simulink model "APPL_PaFaultDetection"  (R2018b)
settings: configuration reference "CodeConfig_10_ms" (kept outside this file)
undefined symbols (not defined in the file): CAL_LockErrNoTime_30ms, CAL_ManualSwValid_90s, CAL_MotorHallInvalid_2s, CAL_MotorMaxRunTime_60s, CAL_MotorRelayErr_2s, CAL_MotorStall_750ms, D_DrSoftStopDef_B, D_DrSoftStopDef_F, D_DrSoftStopDef_H, D_DrSoftStopDef_L, D_Relay_DownBackFault, D_Relay_UpFrontFault, D_StallCurrent, enSeatMoveCmd, FALSE, TRUE
libraries: DareLib x91, simulink x2
(part 3 of 4)

== stateflow chart APPL_PaFaultDetection/LogicCtrl/HallError/HallErrorDetection ==
  note: #后期需要增加2F诊断判断20230510
  state MotorHallDetect
    state HeightHallError [parallel] [commented out]
      state Judge [commented out]
        ex:
        HeightHallTimer = 0;
        (default) -> (junction 286) [commented out]
        MotorHallDetect.HeightHallError.Judge -> (junction 286) [commented out]
        (junction 286) -> (junction 373) [commented out] : /*2s超时检测*/
            | [CAL_MotorHallInvalid_2s > HeightHallTimer]
        (junction 373) -> (junction 365) [commented out]
        (junction 286) -> (junction 262) [commented out] : {HeightHallTimer = CAL_MotorHallInvalid_2s;
            | HeightHallFault = 1;
            | Desc_HeightHallDTC = 1;}
        (junction 365) -> (junction 354) [commented out] : /* 粘连或无电机动作 */
            | [MtrCtrlFault_HeightUpVolt == MtrCtrlFault_HeightDownVolt ...
            | || enSeatMoveCmd.EN_NULL == MtrCtrlFault_HeightMotorCmd]
        (junction 365) -> (junction 381) [commented out] : {HeightHallTimer ++;}
        (junction 354) -> (junction 362) [commented out] : {HeightHallTimer = 0;}
        (junction 381) -> (junction 262) [commented out]
        (junction 362) -> (junction 381) [commented out]
        (junction 262) -> (junction 374) [commented out]
        (junction 374) -> (junction 261) [commented out] : /*霍尔计数变化*/
            | [hasChanged(MtrCtrlFault_HeightHallCnt)]
        (junction 374) -> (junction 357) [commented out]
        (junction 261) -> (junction 260) [commented out] : {HeightHallTimer = 0;
            | HeightHallFault = 0;
            | Desc_HeightHallDTC = 0;}
        (junction 260) -> (junction 357) [commented out]
      state Normal [commented out]
        en:
        HeightHallFault = 0;
      state Init [commented out]
        en:
        HeightHallFault = 0;
        Desc_HeightHallDTC = 0;
      (default) -> MotorHallDetect.HeightHallError.Normal [commented out]
      MotorHallDetect.HeightHallError.Normal -> MotorHallDetect.HeightHallError.Judge [commented out] : /*有调节动作*/
          | [enSeatMoveCmd.EN_NULL != MtrCtrlFault_HeightMotorCmd]
      MotorHallDetect.HeightHallError.Judge -> MotorHallDetect.HeightHallError.Normal [commented out] : /* */
          | [(hasChanged(HeightSwCmd) ...
          | || enSeatMoveCmd.EN_NULL == HeightSwCmd) ...
          | && enSeatMoveCmd.EN_NULL == MtrCtrlFault_HeightMotorCmd]
      MotorHallDetect.HeightHallError.Judge -> MotorHallDetect.HeightHallError.Init [commented out] : /* 不满足前置条件 */
          | [FALSE == DrAdj_Dtc_HeatingMat1SC]
      MotorHallDetect.HeightHallError.Init -> MotorHallDetect.HeightHallError.Normal [commented out] : /* 满足前置条件 */
          | [TRUE == DrAdj_Dtc_HeatingMat1SC]
      MotorHallDetect.HeightHallError.Normal -> MotorHallDetect.HeightHallError.Init [commented out] : /* 不满足前置条件 */
          | [FALSE == DrAdj_Dtc_HeatingMat1SC]
    state LengthHallError [parallel]
      settings: executionOrder=1
      state Normal
        en:
        LengthHallFault = 0;
      state Judge
        ex:
        LengthHallTimer = 0;
        (default) -> (junction 320)
        MotorHallDetect.LengthHallError.Judge -> (junction 320) [order 1]
        (junction 320) -> (junction 330) [order 1] : /*2s超时检测*/
            | [CAL_MotorHallInvalid_2s > LengthHallTimer]
        (junction 320) -> (junction 321) [order 2] : {LengthHallTimer = CAL_MotorHallInvalid_2s;
            | LengthHallFault = 1;
            | Desc_LengthHallDTC = 1;}
        (junction 330) -> (junction 401)
        (junction 401) -> (junction 382) [order 1] : /*粘连或无电机动作*/
            | [MtrCtrlFault_LengthForwardVolt == MtrCtrlFault_LengthBackwardVolt ...
            | || enSeatMoveCmd.EN_NULL == MtrCtrlFault_LengthMotorCmd]
        (junction 401) -> (junction 350) [order 2] : {LengthHallTimer ++;}
        (junction 382) -> (junction 372) : {LengthHallTimer = 0;}
        (junction 350) -> (junction 321)
        (junction 372) -> (junction 350)
        (junction 321) -> (junction 335)
        (junction 335) -> (junction 322) [order 1] : /*霍尔计数变化*/
            | [hasChanged(MtrCtrlFault_LengthHallCnt)]
        (junction 335) -> (junction 336) [order 2]
        (junction 322) -> (junction 323) : {LengthHallTimer = 0;
            | LengthHallFault = 0;
            | Desc_LengthHallDTC = 0;}
        (junction 323) -> (junction 336)
        (junction 336) -> (junction 361)
      state Init
        en:
        LengthHallFault = 0;
        Desc_LengthHallDTC = 0;
      (default) -> MotorHallDetect.LengthHallError.Normal
      MotorHallDetect.LengthHallError.Normal -> MotorHallDetect.LengthHallError.Judge [order 2] : /*有调节动作*/
          | [enSeatMoveCmd.EN_NULL != MtrCtrlFault_LengthMotorCmd]
      MotorHallDetect.LengthHallError.Judge -> MotorHallDetect.LengthHallError.Normal [order 2] : /*无调节动作*/
          | [(hasChanged(LengthSwCmd) ...
          | || enSeatMoveCmd.EN_NULL == LengthSwCmd) ...
          | && enSeatMoveCmd.EN_NULL == MtrCtrlFault_LengthMotorCmd]
      MotorHallDetect.LengthHallError.Judge -> MotorHallDetect.LengthHallError.Init [order 1] : /* 不满足前置条件 */
          | [FALSE == DrAdj_Dtc_HeatingMat1SC]
      MotorHallDetect.LengthHallError.Init -> MotorHallDetect.LengthHallError.Normal : /* 满足前置条件 */
          | [TRUE == DrAdj_Dtc_HeatingMat1SC]
      MotorHallDetect.LengthHallError.Normal -> MotorHallDetect.LengthHallError.Init [order 1] : /* 不满足前置条件 */
          | [FALSE == DrAdj_Dtc_HeatingMat1SC]
    state BackHallError [parallel]
      settings: executionOrder=2
      state Judge
        ex:
        BackHallTimer = 0;
        (default) -> (junction 398)
        MotorHallDetect.BackHallError.Judge -> (junction 398) [order 1]
        (junction 398) -> (junction 393) [order 1] : /*2s超时检测*/
            | [CAL_MotorHallInvalid_2s > BackHallTimer]
        (junction 398) -> (junction 387) [order 2] : {BackHallTimer = CAL_MotorHallInvalid_2s;
            | BackHallFault = 1;
            | Desc_BackHallDTC = 1;}
        (junction 393) -> (junction 367)
        (junction 367) -> (junction 355) [order 1] : /*粘连或无电机动作*/
            | [MtrCtrlFault_BackForwardVolt == MtrCtrlFault_BackBackwardVolt ...
            | || enSeatMoveCmd.EN_NULL == MtrCtrlFault_BackMotorCmd]
        (junction 367) -> (junction 391) [order 2] : {BackHallTimer ++;}
        (junction 355) -> (junction 390) : {BackHallTimer = 0;}
        (junction 391) -> (junction 387)
        (junction 390) -> (junction 391)
        (junction 387) -> (junction 370)
        (junction 370) -> (junction 347) [order 1] : /*霍尔计数变化*/
            | [hasChanged(MtrCtrlFault_BackHallCnt)]
        (junction 370) -> (junction 377) [order 2]
        (junction 347) -> (junction 399) : {BackHallTimer = 0;
            | BackHallFault = 0;
            | Desc_BackHallDTC = 0;}
        (junction 399) -> (junction 377)
        (junction 377) -> (junction 344)
      state Normal
        en:
        BackHallFault = 0;
      state Init
        en:
        BackHallFault = 0;
        Desc_BackHallDTC = 0;
      (default) -> MotorHallDetect.BackHallError.Normal
      MotorHallDetect.BackHallError.Normal -> MotorHallDetect.BackHallError.Judge [order 2] : /*有调节动作*/
          | [enSeatMoveCmd.EN_NULL != MtrCtrlFault_BackMotorCmd]
      MotorHallDetect.BackHallError.Judge -> MotorHallDetect.BackHallError.Normal [order 2] : /*无调节动作*/
          | [(hasChanged(BackSwCmd) ...
          | || enSeatMoveCmd.EN_NULL == BackSwCmd) ...
          | && enSeatMoveCmd.EN_NULL == MtrCtrlFault_BackMotorCmd]
      MotorHallDetect.BackHallError.Judge -> MotorHallDetect.BackHallError.Init [order 1] : /* 不满足前置条件 */
          | [FALSE == DrAdj_Dtc_HeatingMat1SC]
      MotorHallDetect.BackHallError.Init -> MotorHallDetect.BackHallError.Normal : /* 满足前置条件 */
          | [TRUE == DrAdj_Dtc_HeatingMat1SC]
      MotorHallDetect.BackHallError.Normal -> MotorHallDetect.BackHallError.Init [order 1] : /* 不满足前置条件 */
          | [FALSE == DrAdj_Dtc_HeatingMat1SC]
    state FrontHallError3 [parallel] [commented out]
      state Judge [commented out]
        ex:
        FrontHallTimer = 0;
        (default) -> (junction 277) [commented out]
        MotorHallDetect.FrontHallError3.Judge -> (junction 277) [commented out]
        (junction 277) -> (junction 278) [commented out] : /*2s超时检测*/
            | [CAL_MotorHallInvalid_2s > FrontHallTimer]
        (junction 277) -> (junction 281) [commented out] : {FrontHallTimer = CAL_MotorHallInvalid_2s;
            | FrontHallFault = 1;
            | Desc_FrontHallDTC = 1;}
        (junction 278) -> (junction 279) [commented out]
        (junction 279) -> (junction 280) [commented out] : /*粘连或无电机动作*/
            | [MtrCtrlFault_FrontUpVolt == MtrCtrlFault_FrontDownVolt ...
            | || enSeatMoveCmd.EN_NULL == MtrCtrlFault_FrontMotorCmd]
        (junction 279) -> (junction 282) [commented out] : {FrontHallTimer ++;}
        (junction 280) -> (junction 283) [commented out] : {FrontHallTimer = 0;}
        (junction 282) -> (junction 281) [commented out]
        (junction 283) -> (junction 282) [commented out]
        (junction 281) -> (junction 284) [commented out]
        (junction 284) -> (junction 285) [commented out] : /*霍尔计数变化*/
            | [hasChanged(MtrCtrlFault_FrontHallCnt)]
        (junction 284) -> (junction 287) [commented out]
        (junction 285) -> (junction 288) [commented out] : {FrontHallTimer = 0;
            | FrontHallFault = 0;
            | Desc_FrontHallDTC = 0;}
        (junction 288) -> (junction 287) [commented out]
        (junction 287) -> (junction 289) [commented out]
      state Normal [commented out]
        en:
        FrontHallFault = 0;
      state Init [commented out]
        en:
        FrontHallFault = 0;
        Desc_FrontHallDTC = 0;
      (default) -> MotorHallDetect.FrontHallError3.Normal [commented out]
      MotorHallDetect.FrontHallError3.Normal -> MotorHallDetect.FrontHallError3.Judge [commented out] : /*有调节动作*/
          | [enSeatMoveCmd.EN_NULL != MtrCtrlFault_FrontMotorCmd ...
          |  && EN_DrTwelveWayMotor == MtrCtrlFault_DrAdjustCfg]
      MotorHallDetect.FrontHallError3.Judge -> MotorHallDetect.FrontHallError3.Normal [commented out] : /*无调节动作*/
          | [((hasChanged(FrontSwCmd) ...
          | || enSeatMoveCmd.EN_NULL == FrontSwCmd) ...
          | && enSeatMoveCmd.EN_NULL == MtrCtrlFault_FrontMotorCmd) ...
          | || EN_DrTwelveWayMotor != MtrCtrlFault_DrAdjustCfg]
      MotorHallDetect.FrontHallError3.Init -> MotorHallDetect.FrontHallError3.Normal [commented out] : /* 满足前置条件 */
          | [TRUE == DrAdj_Dtc_HeatingMat1SC]
      MotorHallDetect.FrontHallError3.Judge -> MotorHallDetect.FrontHallError3.Init [commented out] : /* 不满足前置条件 */
          | [FALSE == DrAdj_Dtc_HeatingMat1SC ...
          | || EN_DrTwelveWayMotor != MtrCtrlFault_DrAdjustCfg]
      MotorHallDetect.FrontHallError3.Normal -> MotorHallDetect.FrontHallError3.Init [commented out] : /* 不满足前置条件 */
          | [FALSE == DrAdj_Dtc_HeatingMat1SC]
  state Init
    en:
    HeightHallFault = 0;
    HeightHallTimer = 0;
    Desc_HeightHallDTC = 0;
    LengthHallFault = 0;
    LengthHallTimer = 0;
    Desc_LengthHallDTC = 0;
    BackHallFault = 0;
    BackHallTimer = 0;
    Desc_BackHallDTC = 0;
    FrontHallFault = 0;
    FrontHallTimer = 0;
    Desc_FrontHallDTC = 0;
  (default) -> Init
  Init -> MotorHallDetect : /* 有记忆功能 且非不可调节配置 */
      | [TRUE == MtrCtrlFault_DrMemoryCfg ...
      | && TRUE == MtrCtrlFault_DrAdjustCfg]
  MotorHallDetect -> Init : /* 无记忆功能 ||不可调节配置 */
      | [TRUE != MtrCtrlFault_DrMemoryCfg ...
      | || TRUE != MtrCtrlFault_DrAdjustCfg]
  data: HeightSwCmd input; LengthSwCmd input; BackSwCmd input; FrontSwCmd input; MtrCtrlFault_HeightUpVolt input; MtrCtrlFault_HeightDownVolt input; MtrCtrlFault_LengthForwardVolt input; MtrCtrlFault_LengthBackwardVolt input; Desc_HeightHallDTC output uint8 =0; Desc_LengthHallDTC output uint8 =0; Desc_BackHallDTC output uint8 =0; Desc_FrontHallDTC output uint8 =0; MtrCtrlFault_BackForwardVolt input; MtrCtrlFault_BackBackwardVolt input; MtrCtrlFault_FrontUpVolt input; MtrCtrlFault_FrontDownVolt input; HeightHallFault output uint8; MtrCtrlFault_HeightHallCnt input; MtrCtrlFault_LengthHallCnt input; MtrCtrlFault_BackHallCnt input; MtrCtrlFault_FrontHallCnt input; MtrCtrlFault_HeightMotorCmd input; MtrCtrlFault_LengthMotorCmd input; MtrCtrlFault_BackMotorCmd input; MtrCtrlFault_FrontMotorCmd input; HeightHallTimer local uint8; CAL_MotorHallInvalid_2s parameter; LengthHallTimer local uint8; LengthHallFault output uint8; BackHallTimer local uint8; BackHallFault output uint8; FrontHallTimer local uint8; FrontHallFault output uint8; FALSE parameter; TRUE parameter; DrAdj_Dtc_HeatingMat1SC local boolean =1; MtrCtrlFault_DrAdjustCfg input; MtrCtrlFault_DrMemoryCfg input

== stateflow chart APPL_PaFaultDetection/LogicCtrl/StallError/StallErrorDetection ==
  state HeightStallError [parallel] [commented out]
    state Judge [commented out]
      ex:
      HeightStallTimer = 0;
      HeightStallNoTimer = 0;
      (default) -> (junction 16) [commented out]
      HeightStallError.Judge -> (junction 16) [commented out]
      (junction 16) -> (junction 19) [commented out] : /*达到堵转电流 且无霍尔变化 */
          | [LocalHeightHallCnt == MtrCtrlFault_HeightHallCnt]
      (junction 19) -> (junction 187) [commented out] : [1 == MtrCtrlFault_HeightCurrentOverFlag]
      (junction 187) -> (junction 194) [commented out] : [CurrentOverTimer1 < 255]
      (junction 16) -> (junction 30) [commented out] : {HeightStallTimer = 0;
          | CurrentOverTimer1 = 0;}
      (junction 19) -> (junction 191) [commented out] : {CurrentOverTimer1 = 0;}
      (junction 187) -> (junction 189) [commented out]
      (junction 194) -> (junction 196) [commented out] : /* 高度大电流计时器 - 启动电压不超过30ms*/
          | {CurrentOverTimer1 ++;}
      (junction 189) -> (junction 191) [commented out]
      (junction 196) -> (junction 189) [commented out]
      (junction 191) -> (junction 21) [commented out]
      (junction 21) -> (junction 23) [commented out] : /*高度的堵转条件检测*/
          | [HeightStallTimer > CAL_MotorStall_750ms  ...
          | && CurrentOverTimer1 > 20]
      (junction 21) -> (junction 28) [commented out] : /* 高度无霍尔计时器*/
          | {HeightStallTimer ++;}
      (junction 23) -> (junction 26) [commented out] : {HeightStallFault = 1;
          | HeightStallTimer = CAL_MotorStall_750ms;
          | HeightStallNoTimer = 0;}
      (junction 28) -> (junction 30) [commented out]
      (junction 26) -> (junction 28) [commented out]
      (junction 30) -> (junction 43) [commented out] : {LocalHeightHallCnt = MtrCtrlFault_HeightHallCnt;}
      (junction 43) -> (junction 161) [commented out] : /*无调节动作 同时没有本地开关*/
          | [enSeatMoveCmd.EN_NULL == MtrCtrlFault_HeightMotorCmd ...
          | && enSeatMoveCmd.EN_NULL == HeightSwCmd]
      (junction 43) -> (junction 169) [commented out]
      (junction 161) -> (junction 163) [commented out] : {HeightStallNoTimer++;}
      (junction 163) -> (junction 169) [commented out]
      (junction 169) -> (junction 172) [commented out]
    state Normal [commented out]
      en:
      HeightStallFault = 0;
      CurrentOverTimer1 = 0;
    (default) -> HeightStallError.Normal [commented out]
    HeightStallError.Normal -> HeightStallError.Judge [commented out] : /*有调节动作*/
        | [enSeatMoveCmd.EN_NULL != MtrCtrlFault_HeightMotorCmd ...
        | && MtrCtrl_PowerModeStatus != enIgnSts.eCrank]
    HeightStallError.Judge -> HeightStallError.Normal [commented out] : /* 超过故障计时 或按键变化 */
        | [CAL_LockErrNoTime_30ms < HeightStallNoTimer ...
        | || hasChanged(HeightSwCmd) ...
        | || MtrCtrl_PowerModeStatus == enIgnSts.eCrank]
  state LengthStallError [parallel]
    settings: executionOrder=1
    state Judge
      ex:
      LengthStallTimer = 0;
      LengthStallNoTimer = 0;
      (default) -> (junction 53)
      LengthStallError.Judge -> (junction 53) [order 1]
      (junction 53) -> (junction 57) [order 1] : /*达到堵转电流 且无霍尔变化*/
          | [LocalLengthHallCnt == MtrCtrlFault_LengthHallCnt]
      (junction 57) -> (junction 210) [order 1] : [1 == MtrCtrlFault_LengthCurrentOverFlag]
      (junction 210) -> (junction 212) [order 1] : [CurrentOverTimer2 < 255]
      (junction 53) -> (junction 68) [order 2] : {LengthStallTimer = 0;
          | CurrentOverTimer2 = 0;}
      (junction 57) -> (junction 208) [order 2] : {CurrentOverTimer2 = 0;}
      (junction 210) -> (junction 216) [order 2]
      (junction 212) -> (junction 214) : /* 纵向大电流计时器*/
          | {CurrentOverTimer2 ++;}
      (junction 216) -> (junction 208)
      (junction 214) -> (junction 216)
      (junction 208) -> (junction 60)
      (junction 60) -> (junction 52) [order 1] : /*纵向的堵转条件检测*/
          | [LengthStallTimer > CAL_MotorStall_750ms  ...
          | && CurrentOverTimer2 > 20]
      (junction 60) -> (junction 74) [order 2] : {LengthStallTimer ++;}
      (junction 52) -> (junction 62) : {LengthStallTimer = CAL_MotorStall_750ms;
          | LengthStallFault = 1;
          | LengthStallNoTimer = 0;}
      (junction 74) -> (junction 68)
      (junction 62) -> (junction 74)
      (junction 68) -> (junction 78) : {LocalLengthHallCnt = MtrCtrlFault_LengthHallCnt;}
      (junction 78) -> (junction 80) [order 1] : /*无调节动作 同时没有本地开关*/
          | [enSeatMoveCmd.EN_NULL == MtrCtrlFault_LengthMotorCmd ...
          | && enSeatMoveCmd.EN_NULL == LengthSwCmd]
      (junction 78) -> (junction 70) [order 2]
      (junction 80) -> (junction 72) : {LengthStallNoTimer ++;}
      (junction 72) -> (junction 70)
      (junction 70) -> (junction 64)
    state Normal
      en:
      LengthStallFault = 0;
      CurrentOverTimer2 = 0;
    (default) -> LengthStallError.Normal
    LengthStallError.Normal -> LengthStallError.Judge : /*有调节动作*/
        | [enSeatMoveCmd.EN_NULL != MtrCtrlFault_LengthMotorCmd ...
        | && MtrCtrl_PowerModeStatus != enIgnSts.eCrank]
    LengthStallError.Judge -> LengthStallError.Normal [order 1] : /* 超过故障计时 或按键变化 */
        | [CAL_LockErrNoTime_30ms < LengthStallNoTimer ...
        | || hasChanged(LengthSwCmd) ...
        | || MtrCtrl_PowerModeStatus == enIgnSts.eCrank]
  state BackStallError [parallel]
    settings: executionOrder=2
    state Judge
      ex:
      BackStallTimer = 0;
      BackStallNoTimer = 0;
      (default) -> (junction 87)
      BackStallError.Judge -> (junction 87) [order 1]
      (junction 87) -> (junction 91) [order 1] : /* 无霍尔变化超时检测*/
          | [LocalBackHallCnt == MtrCtrlFault_BackHallCnt]
      (junction 91) -> (junction 223) [order 1] : [1 == MtrCtrlFault_BackCurrentOverFlag]
      (junction 223) -> (junction 228) [order 1] : [CurrentOverTimer3 < 255]
      (junction 87) -> (junction 102) [order 2] : {BackStallTimer = 0;
          | CurrentOverTimer3 = 0;}
      (junction 91) -> (junction 231) [order 2] : {CurrentOverTimer3 = 0;}
      (junction 223) -> (junction 229) [order 2]
      (junction 228) -> (junction 222) : /* 靠背大电流计时器*/
          | {CurrentOverTimer3 ++;}
      (junction 229) -> (junction 231)
      (junction 222) -> (junction 229)
      (junction 231) -> (junction 94)
      (junction 94) -> (junction 86) [order 1] : /*靠背的堵转条件检测*/
          | [BackStallTimer > CAL_MotorStall_750ms  ...
          | && CurrentOverTimer3 > 20]
      (junction 94) -> (junction 108) [order 2] : {BackStallTimer ++;}
      (junction 86) -> (junction 96) : {BackStallTimer = CAL_MotorStall_750ms;
          | BackStallFault = 1;
          | BackStallNoTimer = 0;}
      (junction 108) -> (junction 102)
      (junction 96) -> (junction 108)
      (junction 102) -> (junction 112) : {LocalBackHallCnt = MtrCtrlFault_BackHallCnt;}
      (junction 112) -> (junction 114) [order 1] : /*无调节动作 同时没有本地开关*/
          | [enSeatMoveCmd.EN_NULL == MtrCtrlFault_BackMotorCmd ...
          | && enSeatMoveCmd.EN_NULL == BackSwCmd]
      (junction 112) -> (junction 104) [order 2]
      (junction 114) -> (junction 106) : {BackStallNoTimer ++;}
      (junction 106) -> (junction 104)
      (junction 104) -> (junction 98)
    state Normal
      en:
      BackStallFault = 0;
      CurrentOverTimer3 = 0;
    (default) -> BackStallError.Normal
    BackStallError.Normal -> BackStallError.Judge : /*有调节动作*/
        | [enSeatMoveCmd.EN_NULL != MtrCtrlFault_BackMotorCmd ...
        | && MtrCtrl_PowerModeStatus != enIgnSts.eCrank]
    BackStallError.Judge -> BackStallError.Normal [order 1] : /* 超过故障计时 或按键变化 */
        | [CAL_LockErrNoTime_30ms < BackStallNoTimer ...
        | || hasChanged(BackSwCmd) ...
        | || MtrCtrl_PowerModeStatus == enIgnSts.eCrank]
  state FrontStallError [parallel] [commented out]
    state Judge [commented out]
      ex:
      FrontStallTimer = 0;
      (default) -> (junction 121) [commented out]
      FrontStallError.Judge -> (junction 121) [commented out]
      (junction 121) -> (junction 125) [commented out] : /*达到堵转电流 且无霍尔变化*/
          | [1 == MtrCtrlFault_FrontCurrentOverFlag && LocalFrontHallCnt == MtrCtrlFault_FrontHallCnt]
      (junction 121) -> (junction 136) [commented out] : {FrontStallTimer = 0;}
      (junction 125) -> (junction 128) [commented out] : {FrontStallTimer ++;
          | FrontStallNoTimer = 0;}
      (junction 128) -> (junction 120) [commented out] : /*超时检测*/
          | [CAL_MotorStall_750ms <= FrontStallTimer]
      (junction 128) -> (junction 142) [commented out]
      (junction 120) -> (junction 130) [commented out] : {FrontStallTimer = CAL_MotorStall_750ms;
          | FrontStallFault = 1;}
      (junction 142) -> (junction 136) [commented out]
      (junction 130) -> (junction 142) [commented out]
      (junction 136) -> (junction 146) [commented out] : {LocalFrontHallCnt = MtrCtrlFault_FrontHallCnt;}
      (junction 146) -> (junction 148) [commented out] : /*无调节动作 同时没有本地开关*/
          | [enSeatMoveCmd.EN_NULL == MtrCtrlFault_FrontMotorCmd ...
          | && enSeatMoveCmd.EN_NULL == FrontSwCmd]
      (junction 146) -> (junction 138) [commented out]
      (junction 148) -> (junction 140) [commented out] : {FrontStallNoTimer ++;}
      (junction 140) -> (junction 138) [commented out]
      (junction 138) -> (junction 132) [commented out]
    state Normal [commented out]
      en:
      FrontStallFault = 0;
    (default) -> FrontStallError.Normal [commented out]
    FrontStallError.Normal -> FrontStallError.Judge [commented out] : /*有调节动作*/
        | [enSeatMoveCmd.EN_NULL != MtrCtrlFault_FrontMotorCmd]
    FrontStallError.Judge -> FrontStallError.Normal [commented out] : /* 超过故障计时 或按键变化 */
        | [CAL_LockErrNoTime_30ms < FrontStallNoTimer ...
        | || hasChanged(FrontSwCmd)]
  data: HeightSwCmd input; LengthSwCmd input; BackSwCmd input; HeightStallFault output uint8; FrontSwCmd input; MtrCtrlFault_HeightMotorCmd input; MtrCtrlFault_LengthMotorCmd input; MtrCtrlFault_BackMotorCmd input; MtrCtrlFault_FrontMotorCmd input; HeightStallTimer local uint8; CAL_MotorStall_750ms parameter; LengthStallTimer local uint8; LengthStallFault output uint8; BackStallTimer local uint8; BackStallFault output uint8; FrontStallTimer local uint8; FrontStallFault output uint8; D_StallCurrent parameter; MtrCtrlFault_HeightCurrentOverFlag input; MtrCtrlFault_LengthCurrentOverFlag input; MtrCtrlFault_BackCurrentOverFlag input; MtrCtrlFault_FrontCurrentOverFlag input; HeightStallNoTimer local uint8; LengthStallNoTimer local uint8; BackStallNoTimer local uint8; FrontStallNoTimer local uint8; CAL_LockErrNoTime_30ms parameter; MtrCtrlFault_HeightHallCnt input; MtrCtrlFault_LengthHallCnt input; MtrCtrlFault_BackHallCnt input; MtrCtrlFault_FrontHallCnt input; LocalLengthHallCnt local uint16; LocalHeightHallCnt local uint16; LocalBackHallCnt local uint16; LocalFrontHallCnt local uint16; MtrCtrl_PowerModeStatus input; CurrentOverTimer1 local uint8; CurrentOverTimer2 local uint8; CurrentOverTimer3 local uint8

== stateflow chart APPL_PaFaultDetection/LogicCtrl/RelayError/MidRelayErrorDetection/CheckMidRelayFault1/RelayFault ==
  state Judge
    ex:
    MidRelayTimer = 0;
    (default) -> (junction 8)
    Judge -> (junction 8) [order 1]
    (junction 8) -> (junction 10) [order 1] : [CAL_MotorRelayErr_2s <= MidRelayTimer]
    (junction 8) -> (junction 14) [order 2] : {MidRelayTimer ++;}
    (junction 10) -> (junction 12) : {MidRelayTimer = CAL_MotorRelayErr_2s;}
    (junction 12) -> (junction 16) [order 1] : [enSeatMoveCmd.EN_UP_FORWARD != MotorCmd ...
        | && FALSE != UpForwardVolt]
    (junction 12) -> (junction 20) [order 2]
    (junction 16) -> (junction 18) : {MidRelayFault = D_Relay_UpFrontFault;}
    (junction 20) -> (junction 23) [order 1] : [enSeatMoveCmd.EN_DN_BACKWARD != MotorCmd ...
        | && FALSE != DownBackwardVolt]
    (junction 20) -> (junction 27) [order 2]
    (junction 23) -> (junction 25) : {MidRelayFault = D_Relay_DownBackFault;}
    (junction 14) -> (junction 27)
    (junction 25) -> (junction 27)
    (junction 18) -> (junction 25)
    (junction 27) -> (junction 31)
  state Normal
    en:
    MidRelayFault = FALSE;
    MidRelayTimer = 0;
  (default) -> Normal
  Normal -> Judge [order 1] : [/*没有输出命令但输出反馈有电压 满足前置条件*/
      | enSeatMoveCmd.EN_NULL == MotorCmd...
      | && (FALSE != UpForwardVolt...
      | || FALSE != DownBackwardVolt)]
  Normal -> Judge [order 2] : [/*输出命令向前/向上命令却有向后/向下电压 */
      | enSeatMoveCmd.EN_UP_FORWARD == MotorCmd...
      | &&  FALSE != DownBackwardVolt]
  Normal -> Judge [order 3] : [/*输出命令向后/向下命令却有向前/向上电压 */
      | enSeatMoveCmd.EN_DN_BACKWARD  == MotorCmd...
      | &&  FALSE != UpForwardVolt]
  Judge -> Normal [order 1] : [/*继电器粘连消失：
      |  1、没有控制开启命令，同时没有电压输出，认为继电器粘连消失
      |  2、控制开启命令，存在对应的电压输出，认为继电器粘连消失*/
      | (enSeatMoveCmd.EN_NULL == MotorCmd...
      | && FALSE == UpForwardVolt...
      | && FALSE == DownBackwardVolt) ...
      | || (enSeatMoveCmd.EN_UP_FORWARD == MotorCmd...
      | && TRUE == UpForwardVolt ...
      | && FALSE == DownBackwardVolt) ...
      | || (enSeatMoveCmd.EN_DN_BACKWARD == MotorCmd ...
      | && FALSE == UpForwardVolt ...
      | && TRUE == DownBackwardVolt) ]
  data: MotorCmd input; UpForwardVolt input; DownBackwardVolt input; MidRelayFault output uint8; CAL_MotorRelayErr_2s parameter; D_Relay_DownBackFault parameter; D_Relay_UpFrontFault parameter; FALSE parameter; TRUE parameter; MidRelayTimer output uint8

== stateflow chart APPL_PaFaultDetection/LogicCtrl/RelayError/MidRelayErrorDetection/CheckMidRelayFault2/RelayFault ==
  state Judge
    ex:
    MidRelayTimer = 0;
    (default) -> (junction 8)
    Judge -> (junction 8) [order 1]
    (junction 8) -> (junction 10) [order 1] : [CAL_MotorRelayErr_2s <= MidRelayTimer]
    (junction 8) -> (junction 14) [order 2] : {MidRelayTimer ++;}
    (junction 10) -> (junction 12) : {MidRelayTimer = CAL_MotorRelayErr_2s;}
    (junction 12) -> (junction 16) [order 1] : [enSeatMoveCmd.EN_UP_FORWARD != MotorCmd ...
        | && FALSE != UpForwardVolt]
    (junction 12) -> (junction 20) [order 2]
    (junction 16) -> (junction 18) : {MidRelayFault = D_Relay_UpFrontFault;}
    (junction 20) -> (junction 23) [order 1] : [enSeatMoveCmd.EN_DN_BACKWARD != MotorCmd ...
        | && FALSE != DownBackwardVolt]
    (junction 20) -> (junction 27) [order 2]
    (junction 23) -> (junction 25) : {MidRelayFault = D_Relay_DownBackFault;}
    (junction 14) -> (junction 27)
    (junction 25) -> (junction 27)
    (junction 18) -> (junction 25)
    (junction 27) -> (junction 31)
  state Normal
    en:
    MidRelayFault = FALSE;
    MidRelayTimer = 0;
  (default) -> Normal
  Normal -> Judge [order 1] : [/*没有输出命令但输出反馈有电压 满足前置条件*/
      | enSeatMoveCmd.EN_NULL == MotorCmd...
      | && (FALSE != UpForwardVolt...
      | || FALSE != DownBackwardVolt)]
  Normal -> Judge [order 2] : [/*输出命令向前/向上命令却有向后/向下电压 */
      | enSeatMoveCmd.EN_UP_FORWARD == MotorCmd...
      | &&  FALSE != DownBackwardVolt]
  Normal -> Judge [order 3] : [/*输出命令向后/向下命令却有向前/向上电压 */
      | enSeatMoveCmd.EN_DN_BACKWARD  == MotorCmd...
      | &&  FALSE != UpForwardVolt]
  Judge -> Normal [order 1] : [/*继电器粘连消失：
      |  1、没有控制开启命令，同时没有电压输出，认为继电器粘连消失
      |  2、控制开启命令，存在对应的电压输出，认为继电器粘连消失*/
      | (enSeatMoveCmd.EN_NULL == MotorCmd...
      | && FALSE == UpForwardVolt...
      | && FALSE == DownBackwardVolt) ...
      | || (enSeatMoveCmd.EN_UP_FORWARD == MotorCmd...
      | && TRUE == UpForwardVolt ...
      | && FALSE == DownBackwardVolt) ...
      | || (enSeatMoveCmd.EN_DN_BACKWARD == MotorCmd ...
      | && FALSE == UpForwardVolt ...
      | && TRUE == DownBackwardVolt) ]
  data: MotorCmd input; UpForwardVolt input; DownBackwardVolt input; MidRelayFault output uint8; CAL_MotorRelayErr_2s parameter; D_Relay_DownBackFault parameter; D_Relay_UpFrontFault parameter; FALSE parameter; TRUE parameter; MidRelayTimer output uint8

== stateflow chart APPL_PaFaultDetection/LogicCtrl/RelayError/MidRelayErrorDetection/CheckMidRelayFault3/RelayFault ==
  state Judge
    ex:
    MidRelayTimer = 0;
    (default) -> (junction 8)
    Judge -> (junction 8) [order 1]
    (junction 8) -> (junction 10) [order 1] : [CAL_MotorRelayErr_2s <= MidRelayTimer]
    (junction 8) -> (junction 14) [order 2] : {MidRelayTimer ++;}
    (junction 10) -> (junction 12) : {MidRelayTimer = CAL_MotorRelayErr_2s;}
    (junction 12) -> (junction 16) [order 1] : [enSeatMoveCmd.EN_UP_FORWARD != MotorCmd ...
        | && FALSE != UpForwardVolt]
    (junction 12) -> (junction 20) [order 2]
    (junction 16) -> (junction 18) : {MidRelayFault = D_Relay_UpFrontFault;}
    (junction 20) -> (junction 23) [order 1] : [enSeatMoveCmd.EN_DN_BACKWARD != MotorCmd ...
        | && FALSE != DownBackwardVolt]
    (junction 20) -> (junction 27) [order 2]
    (junction 23) -> (junction 25) : {MidRelayFault = D_Relay_DownBackFault;}
    (junction 14) -> (junction 27)
    (junction 25) -> (junction 27)
    (junction 18) -> (junction 25)
    (junction 27) -> (junction 31)
  state Normal
    en:
    MidRelayFault = FALSE;
    MidRelayTimer = 0;
  (default) -> Normal
  Normal -> Judge [order 1] : [/*没有输出命令但输出反馈有电压 满足前置条件*/
      | enSeatMoveCmd.EN_NULL == MotorCmd...
      | && (FALSE != UpForwardVolt...
      | || FALSE != DownBackwardVolt)]
  Normal -> Judge [order 2] : [/*输出命令向前/向上命令却有向后/向下电压 */
      | enSeatMoveCmd.EN_UP_FORWARD == MotorCmd...
      | &&  FALSE != DownBackwardVolt]
  Normal -> Judge [order 3] : [/*输出命令向后/向下命令却有向前/向上电压 */
      | enSeatMoveCmd.EN_DN_BACKWARD  == MotorCmd...
      | &&  FALSE != UpForwardVolt]
  Judge -> Normal [order 1] : [/*继电器粘连消失：
      |  1、没有控制开启命令，同时没有电压输出，认为继电器粘连消失
      |  2、控制开启命令，存在对应的电压输出，认为继电器粘连消失*/
      | (enSeatMoveCmd.EN_NULL == MotorCmd...
      | && FALSE == UpForwardVolt...
      | && FALSE == DownBackwardVolt) ...
      | || (enSeatMoveCmd.EN_UP_FORWARD == MotorCmd...
      | && TRUE == UpForwardVolt ...
      | && FALSE == DownBackwardVolt) ...
      | || (enSeatMoveCmd.EN_DN_BACKWARD == MotorCmd ...
      | && FALSE == UpForwardVolt ...
      | && TRUE == DownBackwardVolt) ]
  data: MotorCmd input; UpForwardVolt input; DownBackwardVolt input; MidRelayFault output uint8; CAL_MotorRelayErr_2s parameter; D_Relay_DownBackFault parameter; D_Relay_UpFrontFault parameter; FALSE parameter; TRUE parameter; MidRelayTimer output uint8

== stateflow chart APPL_PaFaultDetection/LogicCtrl/MotorTimeOut/MotorTimeOutDetection ==
  state HeightAdjust [parallel] [commented out]
    state Init [commented out]
      en:
      HeightTimer = 0;
      (default) -> (junction 362) [commented out]
      HeightAdjust.Init -> (junction 362) [commented out]
      (junction 362) -> (junction 365) [commented out] : /* 按键无效 */
          | [FALSE == HeightManualAdjSw]
      (junction 362) -> (junction 369) [commented out]
      (junction 365) -> (junction 367) [commented out] : {HeightTimeOutFlag =FALSE;}
      (junction 367) -> (junction 369) [commented out]
      (junction 369) -> (junction 372) [commented out]
    state Action [commented out]
      (default) -> (junction 25) [commented out]
      HeightAdjust.Action -> (junction 25) [commented out]
      (junction 25) -> (junction 26) [commented out] : [HeightTimer < CAL_MotorMaxRunTime_60s]
      (junction 25) -> (junction 27) [commented out] : {HeightTimeOutFlag =TRUE;}
      (junction 26) -> (junction 28) [commented out] : {HeightTimer++;}
      (junction 28) -> (junction 27) [commented out]
      (junction 27) -> (junction 317) [commented out]
    (default) -> HeightAdjust.Init [commented out]
    HeightAdjust.Init -> HeightAdjust.Action [commented out] : [EN_NULL != HeightMotorCmd]
    HeightAdjust.Action -> HeightAdjust.Init [commented out] : [EN_NULL == HeightMotorCmd]
  state VerticalAdjust [parallel]
    settings: executionOrder=1
    state Init
      en:
      LengthTimer = 0;
      (default) -> (junction 383)
      VerticalAdjust.Init -> (junction 383) [order 1]
      (junction 383) -> (junction 378) [order 1] : /* 按键无效 */
          | [FALSE == LengthManualAdjSw]
      (junction 383) -> (junction 385) [order 2]
      (junction 378) -> (junction 381) : {LengthTimeOutFlag = FALSE;}
      (junction 381) -> (junction 385)
      (junction 385) -> (junction 375)
    state Action
      (default) -> (junction 38)
      VerticalAdjust.Action -> (junction 38) [order 1]
      (junction 38) -> (junction 32) [order 1] : [LengthTimer < CAL_MotorMaxRunTime_60s]
      (junction 38) -> (junction 33) [order 2] : {LengthTimeOutFlag = TRUE;}
      (junction 32) -> (junction 40) : {LengthTimer++;}
      (junction 40) -> (junction 33)
      (junction 33) -> (junction 320)
    (default) -> VerticalAdjust.Init
    VerticalAdjust.Init -> VerticalAdjust.Action [order 1] : /*高度、纵向电机没有命令或计时已到*/
        | [EN_NULL != LengthMotorCmd]
    VerticalAdjust.Action -> VerticalAdjust.Init [order 1] : [EN_NULL == LengthMotorCmd]
  state BackAdjust [parallel]
    settings: executionOrder=2
    state Init
      en:
      BackTimer = 0;
      (default) -> (junction 390)
      BackAdjust.Init -> (junction 390) [order 1]
      (junction 390) -> (junction 395) [order 1] : /* 按键无效 */
          | [FALSE == BackManualAdjSw]
      (junction 390) -> (junction 388) [order 2]
      (junction 395) -> (junction 392) : {BackTimeOutFlag = FALSE;}
      (junction 392) -> (junction 388)
      (junction 388) -> (junction 394)
    state Action
      (default) -> (junction 79)
      BackAdjust.Action -> (junction 79) [order 1]
      (junction 79) -> (junction 73) [order 1] : [BackTimer < CAL_MotorMaxRunTime_60s]
      (junction 79) -> (junction 74) [order 2] : {BackTimeOutFlag = TRUE;}
      (junction 73) -> (junction 81) : {BackTimer++;}
      (junction 81) -> (junction 74)
      (junction 74) -> (junction 340)
    (default) -> BackAdjust.Init
    BackAdjust.Init -> BackAdjust.Action [order 1] : /*高度、纵向、前部电机没有命令或计时已到*/
        | [EN_NULL != BackMotorCmd]
    BackAdjust.Action -> BackAdjust.Init [order 1] : [EN_NULL == BackMotorCmd]
  state FrontAngleAdjust [parallel] [commented out]
    state Init [commented out]
      en:
      FrontTimer = 0;
      (default) -> (junction 406) [commented out]
      FrontAngleAdjust.Init -> (junction 406) [commented out]
      (junction 406) -> (junction 401) [commented out] : /* 按键无效 */
          | [FALSE == FrontManualAdjSw]
      (junction 406) -> (junction 403) [commented out]
      (junction 401) -> (junction 400) [commented out] : {FrontTimeOutFlag = FALSE;}
      (junction 400) -> (junction 403) [commented out]
      (junction 403) -> (junction 399) [commented out]
    state Action [commented out]
      (default) -> (junction 103) [commented out]
      FrontAngleAdjust.Action -> (junction 103) [commented out]
      (junction 103) -> (junction 109) [commented out] : [FrontTimer < CAL_MotorMaxRunTime_60s]
      (junction 103) -> (junction 101) [commented out] : {FrontTimeOutFlag = TRUE;}
      (junction 109) -> (junction 98) [commented out] : {FrontTimer++;}
      (junction 98) -> (junction 101) [commented out]
      (junction 101) -> (junction 352) [commented out]
    FrontAngleAdjust.Init -> FrontAngleAdjust.Action [commented out] : /*高度、纵向电机没有命令或计时已到*/
        | [EN_NULL != FrontMotorCmd]
    FrontAngleAdjust.Action -> FrontAngleAdjust.Init [commented out] : [EN_NULL == FrontMotorCmd]
  (default) -> FrontAngleAdjust.Init [commented out]
  data: HeightMotorCmd input; LengthMotorCmd input; BackMotorCmd input; FrontMotorCmd input; EN_NULL input; BackTimer local uint16; FrontTimer local uint16; HeightTimer local uint16; LengthTimer local uint16; HeightTimeOutFlag output uint8; LengthTimeOutFlag output uint8; BackTimeOutFlag output uint8; FrontTimeOutFlag output uint8; CAL_MotorMaxRunTime_60s parameter; TRUE parameter; FALSE parameter; HeightManualAdjSw input; LengthManualAdjSw input; BackManualAdjSw input; FrontManualAdjSw input

== stateflow chart APPL_PaFaultDetection/LogicCtrl/SoftStopPoint/SoftStopPointDetection ==
  state InputData [parallel]
    en:
    du:
    HeightSoftStopBufCnt = MtrCtrlFault_HeightSoftStopCnt;
    LengthSoftStopBufCnt = MtrCtrlFault_LengthSoftStopCnt;
    BackSoftStopBufCnt = MtrCtrlFault_BackSoftStopCnt;
    FrontSoftStopBufCnt = MtrCtrlFault_FrontSoftStopCnt;
    settings: executionOrder=1
  state DrAdj_SetHeightSoftStopCnt(Cnt) [function]
  state DrAdj_SetLengthSoftStopCnt(Cnt) [function]
  state HeightSoft [parallel] [commented out]
    state LeftUpFront [commented out]
      (default) -> (junction 55) [commented out]
      HeightSoft.LeftUpFront -> (junction 55) [commented out]
      (junction 55) -> (junction 58) [commented out] : {HeightSoftStopFault = enSeatMoveCmd.EN_NULL;}
      (junction 58) -> (junction 60) [commented out] : /* 超过最大软止点 */
          | [MtrCtrlFault_HeightHallCnt >= (MtrCtrlFault_HeightStopPosi + MtrCtrlFault_HeightMotorSize - D_DrSoftStopDef_H)]
      (junction 58) -> (junction 69) [commented out]
      (junction 60) -> (junction 67) [commented out] : {HeightSoftStopBufCnt += 1;
          | HeightSoftStopFault = enSeatMoveCmd.EN_UP_FORWARD;
          | DrAdj_SetHeightSoftStopCnt(HeightSoftStopBufCnt);}
      (junction 67) -> (junction 69) [commented out]
      (junction 69) -> (junction 87) [commented out]
    state Init [commented out]
      (default) -> (junction 91) [commented out]
      HeightSoft.Init -> (junction 91) [commented out]
      (junction 91) -> (junction 94) [commented out] : /*超过计数无故障 */
          | [HeightSoftStopBufCnt >= MtrCtrlFault_MotorSoftStopCntMax]
      (junction 91) -> (junction 98) [commented out]
      (junction 94) -> (junction 96) [commented out] : {HeightSoftStopFault = enSeatMoveCmd.EN_NULL;}
      (junction 96) -> (junction 98) [commented out]
      (junction 98) -> (junction 101) [commented out]
    state RightDnBack [commented out]
      (default) -> (junction 82) [commented out]
      HeightSoft.RightDnBack -> (junction 82) [commented out]
      (junction 82) -> (junction 85) [commented out] : {HeightSoftStopFault = enSeatMoveCmd.EN_NULL;}
      (junction 85) -> (junction 83) [commented out] : /* 超过最小软止点 */
          | [MtrCtrlFault_HeightHallCnt <= (MtrCtrlFault_HeightStopPosi + D_DrSoftStopDef_H)]
      (junction 85) -> (junction 79) [commented out]
      (junction 83) -> (junction 78) [commented out] : {HeightSoftStopBufCnt += 1;
          | HeightSoftStopFault = enSeatMoveCmd.EN_DN_BACKWARD;
          | DrAdj_SetHeightSoftStopCnt(HeightSoftStopBufCnt);}
      (junction 78) -> (junction 79) [commented out]
      (junction 79) -> (junction 89) [commented out]
    (default) -> HeightSoft.Init [commented out]
    HeightSoft.Init -> HeightSoft.RightDnBack [commented out] : /* 已学习硬止点
        | 软止点计数小于 最大值
        | 有控制指令 */
        | [0 != MtrCtrlFault_HeightStopPosi ...
        | && 0xFFFF != MtrCtrlFault_HeightStopPosi ...
        | && HeightSoftStopBufCnt < MtrCtrlFault_MotorSoftStopCntMax ...
        | && MtrCtrlFault_HeightMotorCmd == enSeatMoveCmd.EN_DN_BACKWARD ...
        | && HeightSoftStopFault != enSeatMoveCmd.EN_DN_BACKWARD]
    HeightSoft.Init -> HeightSoft.LeftUpFront [commented out] : /* 已学习硬止点
        | 软止点计数小于 最大值
        | 有控制指令 */
        | [0 != MtrCtrlFault_HeightStopPosi ...
        | && 0xFFFF != MtrCtrlFault_HeightStopPosi ...
        | && HeightSoftStopBufCnt < MtrCtrlFault_MotorSoftStopCntMax ...
        | && MtrCtrlFault_HeightMotorCmd == enSeatMoveCmd.EN_UP_FORWARD ...
        | && HeightSoftStopFault != enSeatMoveCmd.EN_UP_FORWARD]
    HeightSoft.LeftUpFront -> HeightSoft.Init [commented out] : /*无控制指令 */
        | [MtrCtrlFault_HeightMotorCmd == enSeatMoveCmd.EN_NULL ...
        | || HeightSoftStopFault == enSeatMoveCmd.EN_UP_FORWARD]
    HeightSoft.RightDnBack -> HeightSoft.Init [commented out] : /*无控制指令 */
        | [MtrCtrlFault_HeightMotorCmd == enSeatMoveCmd.EN_NULL ...
        | || HeightSoftStopFault == enSeatMoveCmd.EN_DN_BACKWARD]
  state DrAdj_SetBackSoftStopCnt(Cnt) [function]
  state DrAdj_SetFrontSoftStopCnt(Cnt) [function]
  state LengthSoft [parallel]
    settings: executionOrder=2
    state LeftUpFront
      (default) -> (junction 124)
      LengthSoft.LeftUpFront -> (junction 124) [order 1]
      (junction 124) -> (junction 129) : {LengthSoftStopFault = enSeatMoveCmd.EN_NULL;}
      (junction 129) -> (junction 125) [order 1] : /* 超过最大软止点 */
          | [MtrCtrlFault_LengthHallCnt >= (MtrCtrlFault_LengthStopPosi + MtrCtrlFault_LengthMotorSize - D_DrSoftStopDef_L)]
      (junction 129) -> (junction 120) [order 2]
      (junction 125) -> (junction 119) : {LengthSoftStopBufCnt += 1;
          | LengthSoftStopFault = enSeatMoveCmd.EN_UP_FORWARD;
          | DrAdj_SetLengthSoftStopCnt(LengthSoftStopBufCnt);}
      (junction 119) -> (junction 120)
      (junction 120) -> (junction 145)
    state Init
      (default) -> (junction 143)
      LengthSoft.Init -> (junction 143) [order 1]
      (junction 143) -> (junction 136) [order 1] : /*超过计数无故障 */
          | [LengthSoftStopBufCnt >= MtrCtrlFault_MotorSoftStopCntMax]
      (junction 143) -> (junction 135) [order 2]
      (junction 136) -> (junction 149) : {LengthSoftStopFault = enSeatMoveCmd.EN_NULL;}
      (junction 149) -> (junction 135)
      (junction 135) -> (junction 138)
    state RightDnBack
      (default) -> (junction 103)
      LengthSoft.RightDnBack -> (junction 103) [order 1]
      (junction 103) -> (junction 111) : {LengthSoftStopFault = enSeatMoveCmd.EN_NULL;}
      (junction 111) -> (junction 112) [order 1] : /* 超过最小软止点 */
          | [MtrCtrlFault_LengthHallCnt <= (MtrCtrlFault_LengthStopPosi + D_DrSoftStopDef_L)]
      (junction 111) -> (junction 108) [order 2]
      (junction 112) -> (junction 105) : {LengthSoftStopBufCnt += 1;
          | LengthSoftStopFault = enSeatMoveCmd.EN_DN_BACKWARD;
          | DrAdj_SetLengthSoftStopCnt(LengthSoftStopBufCnt);}
      (junction 105) -> (junction 108)
      (junction 108) -> (junction 140)
    (default) -> LengthSoft.Init
    LengthSoft.Init -> LengthSoft.RightDnBack [order 2] : /* 已学习硬止点
        | 软止点计数小于 最大值
        | 有控制指令 */
        | [0 != MtrCtrlFault_LengthStopPosi ...
        | && 0xFFFF != MtrCtrlFault_LengthStopPosi ...
        | && LengthSoftStopBufCnt < MtrCtrlFault_MotorSoftStopCntMax ...
        | && MtrCtrlFault_LengthMotorCmd == enSeatMoveCmd.EN_DN_BACKWARD ...
        | && LengthSoftStopFault != enSeatMoveCmd.EN_DN_BACKWARD]
    LengthSoft.Init -> LengthSoft.LeftUpFront [order 1] : /* 已学习硬止点
        | 软止点计数小于 最大值
        | 有控制指令 */
        | [0 != MtrCtrlFault_LengthStopPosi ...
        | && 0xFFFF != MtrCtrlFault_LengthStopPosi ...
        | && LengthSoftStopBufCnt < MtrCtrlFault_MotorSoftStopCntMax ...
        | && MtrCtrlFault_LengthMotorCmd == enSeatMoveCmd.EN_UP_FORWARD ...
        | && LengthSoftStopFault != enSeatMoveCmd.EN_UP_FORWARD]
    LengthSoft.LeftUpFront -> LengthSoft.Init [order 1] : /*无控制指令 */
        | [MtrCtrlFault_LengthMotorCmd == enSeatMoveCmd.EN_NULL ...
        | || LengthSoftStopFault == enSeatMoveCmd.EN_UP_FORWARD]
    LengthSoft.RightDnBack -> LengthSoft.Init [order 1] : /*无控制指令 */
        | [MtrCtrlFault_LengthMotorCmd == enSeatMoveCmd.EN_NULL ...
        | || LengthSoftStopFault == enSeatMoveCmd.EN_DN_BACKWARD]
  state BackSoft [parallel]
    settings: executionOrder=3
    state LeftUpFront
      (default) -> (junction 181)
      BackSoft.LeftUpFront -> (junction 181) [order 1]
      (junction 181) -> (junction 185) : {BackSoftStopFault = enSeatMoveCmd.EN_NULL;}
      (junction 185) -> (junction 156) [order 1] : /* 超过最大软止点 */
          | [MtrCtrlFault_BackHallCnt >= (MtrCtrlFault_BackStopPosi + MtrCtrlFault_BackMotorSize - D_DrSoftStopDef_B)]
      (junction 185) -> (junction 186) [order 2]
      (junction 156) -> (junction 188) : {BackSoftStopBufCnt += 1;
          | BackSoftStopFault = enSeatMoveCmd.EN_UP_FORWARD;
          | DrAdj_SetBackSoftStopCnt(BackSoftStopBufCnt);}
      (junction 188) -> (junction 186)
      (junction 186) -> (junction 163)
    state Init
      (default) -> (junction 170)
      BackSoft.Init -> (junction 170) [order 1]
      (junction 170) -> (junction 158) [order 1] : /*超过计数无故障 */
          | [BackSoftStopBufCnt >= MtrCtrlFault_MotorSoftStopCntMax]
      (junction 170) -> (junction 191) [order 2]
      (junction 158) -> (junction 176) : {BackSoftStopFault = enSeatMoveCmd.EN_NULL;}
      (junction 176) -> (junction 191)
      (junction 191) -> (junction 193)
    state RightDnBack
      (default) -> (junction 184)
      BackSoft.RightDnBack -> (junction 184) [order 1]
      (junction 184) -> (junction 179) : {BackSoftStopFault = enSeatMoveCmd.EN_NULL;}
      (junction 179) -> (junction 177) [order 1] : /* 超过最小软止点 */
          | [MtrCtrlFault_BackHallCnt <= (MtrCtrlFault_BackStopPosi + D_DrSoftStopDef_B)]
      (junction 179) -> (junction 168) [order 2]
      (junction 177) -> (junction 196) : {BackSoftStopBufCnt += 1;
          | BackSoftStopFault = enSeatMoveCmd.EN_DN_BACKWARD;
          | DrAdj_SetBackSoftStopCnt(BackSoftStopBufCnt);}
      (junction 196) -> (junction 168)
      (junction 168) -> (junction 161)
    (default) -> BackSoft.Init
    BackSoft.Init -> BackSoft.RightDnBack [order 2] : /* 已学习硬止点
        | 软止点计数小于 最大值
        | 有控制指令 */
        | [0 != MtrCtrlFault_BackStopPosi ...
        | && 0xFFFF != MtrCtrlFault_BackStopPosi ...
        | && BackSoftStopBufCnt < MtrCtrlFault_MotorSoftStopCntMax ...
        | && MtrCtrlFault_BackMotorCmd == enSeatMoveCmd.EN_DN_BACKWARD ...
        | && BackSoftStopFault != enSeatMoveCmd.EN_DN_BACKWARD]
    BackSoft.Init -> BackSoft.LeftUpFront [order 1] : /* 已学习硬止点
        | 软止点计数小于 最大值
        | 有控制指令 */
        | [0 != MtrCtrlFault_BackStopPosi ...
        | && 0xFFFF != MtrCtrlFault_BackStopPosi ...
        | && BackSoftStopBufCnt < MtrCtrlFault_MotorSoftStopCntMax ...
        | && MtrCtrlFault_BackMotorCmd == enSeatMoveCmd.EN_UP_FORWARD ...
        | && BackSoftStopFault != enSeatMoveCmd.EN_UP_FORWARD]
    BackSoft.LeftUpFront -> BackSoft.Init [order 1] : /*无控制指令 */
        | [MtrCtrlFault_BackMotorCmd == enSeatMoveCmd.EN_NULL ...
        | || BackSoftStopFault == enSeatMoveCmd.EN_UP_FORWARD]
    BackSoft.RightDnBack -> BackSoft.Init [order 1] : /*无控制指令 */
        | [MtrCtrlFault_BackMotorCmd == enSeatMoveCmd.EN_NULL ...
        | || BackSoftStopFault == enSeatMoveCmd.EN_DN_BACKWARD]
  state FrontSoft [parallel] [commented out]
    state LeftUpFront [commented out]
      (default) -> (junction 207) [commented out]
      FrontSoft.LeftUpFront -> (junction 207) [commented out]
      (junction 207) -> (junction 203) [commented out] : {FrontSoftStopFault = enSeatMoveCmd.EN_NULL;}
      (junction 203) -> (junction 228) [commented out] : /* 超过最大软止点 */
          | [MtrCtrlFault_FrontHallCnt >= (MtrCtrlFault_FrontStopPosi + MtrCtrlFault_FrontMotorSize - D_DrSoftStopDef_F)]
      (junction 203) -> (junction 202) [commented out]
      (junction 228) -> (junction 226) [commented out] : {FrontSoftStopBufCnt += 1;
          | FrontSoftStopFault = enSeatMoveCmd.EN_UP_FORWARD;
          | DrAdj_SetFrontSoftStopCnt(FrontSoftStopBufCnt);}
      (junction 226) -> (junction 202) [commented out]
      (junction 202) -> (junction 223) [commented out]
    state Init [commented out]
      (default) -> (junction 218) [commented out]
      FrontSoft.Init -> (junction 218) [commented out]
      (junction 218) -> (junction 230) [commented out] : /*超过计数无故障 */
          | [FrontSoftStopBufCnt >= MtrCtrlFault_MotorSoftStopCntMax]
      (junction 218) -> (junction 250) [commented out]
      (junction 230) -> (junction 212) [commented out] : {FrontSoftStopFault = enSeatMoveCmd.EN_NULL;}
      (junction 212) -> (junction 250) [commented out]
      (junction 250) -> (junction 234) [commented out]
    state RightDnBack [commented out]
      (default) -> (junction 204) [commented out]
      FrontSoft.RightDnBack -> (junction 204) [commented out]
      (junction 204) -> (junction 209) [commented out] : {FrontSoftStopFault = enSeatMoveCmd.EN_NULL;}
      (junction 209) -> (junction 210) [commented out] : /* 超过最小软止点 */
          | [MtrCtrlFault_FrontHallCnt <= (MtrCtrlFault_FrontStopPosi + D_DrSoftStopDef_F)]
      (junction 209) -> (junction 244) [commented out]
      (junction 210) -> (junction 235) [commented out] : {FrontSoftStopBufCnt += 1;
          | FrontSoftStopFault = enSeatMoveCmd.EN_DN_BACKWARD;
          | DrAdj_SetFrontSoftStopCnt(FrontSoftStopBufCnt);}
      (junction 235) -> (junction 244) [commented out]
      (junction 244) -> (junction 222) [commented out]
    (default) -> FrontSoft.Init [commented out]
    FrontSoft.Init -> FrontSoft.RightDnBack [commented out] : /* 已学习硬止点
        | 软止点计数小于 最大值
        | 有控制指令 */
        | [0 != MtrCtrlFault_FrontStopPosi ...
        | && 0xFFFF != MtrCtrlFault_FrontStopPosi ...
        | && FrontSoftStopBufCnt < MtrCtrlFault_MotorSoftStopCntMax ...
        | && MtrCtrlFault_FrontMotorCmd == enSeatMoveCmd.EN_DN_BACKWARD ...
        | && FrontSoftStopFault != enSeatMoveCmd.EN_DN_BACKWARD]
    FrontSoft.Init -> FrontSoft.LeftUpFront [commented out] : /* 已学习硬止点
        | 软止点计数小于 最大值
        | 有控制指令 */
        | [0 != MtrCtrlFault_FrontStopPosi ...
        | && 0xFFFF != MtrCtrlFault_FrontStopPosi ...
        | && FrontSoftStopBufCnt < MtrCtrlFault_MotorSoftStopCntMax ...
        | && MtrCtrlFault_FrontMotorCmd == enSeatMoveCmd.EN_UP_FORWARD ...
        | && FrontSoftStopFault != enSeatMoveCmd.EN_UP_FORWARD]
    FrontSoft.LeftUpFront -> FrontSoft.Init [commented out] : /*无控制指令 */
        | [MtrCtrlFault_FrontMotorCmd == enSeatMoveCmd.EN_NULL ...
        | || FrontSoftStopFault == enSeatMoveCmd.EN_UP_FORWARD]
    FrontSoft.RightDnBack -> FrontSoft.Init [commented out] : /*无控制指令 */
        | [MtrCtrlFault_FrontMotorCmd == enSeatMoveCmd.EN_NULL ...
        | || FrontSoftStopFault == enSeatMoveCmd.EN_DN_BACKWARD]
  data: Cnt function_input; Cnt function_input; Cnt function_input; Cnt function_input; MtrCtrlFault_HeightMotorCmd input; MtrCtrlFault_LengthMotorCmd input; MtrCtrlFault_BackMotorCmd input; MtrCtrlFault_FrontMotorCmd input; MtrCtrlFault_MotorSoftStopCntMax input; MtrCtrlFault_HeightSoftStopCnt input; MtrCtrlFault_LengthSoftStopCnt input; MtrCtrlFault_BackSoftStopCnt input; MtrCtrlFault_FrontSoftStopCnt input; MtrCtrlFault_HeightStopPosi input; MtrCtrlFault_LengthStopPosi input; MtrCtrlFault_BackStopPosi input; MtrCtrlFault_FrontStopPosi input; HeightSoftStopFault output uint8; LengthSoftStopFault output uint8; BackSoftStopFault output uint8; FrontSoftStopFault output uint8; MtrCtrlFault_HeightMotorSize input; MtrCtrlFault_LengthMotorSize input; MtrCtrlFault_BackMotorSize input; MtrCtrlFault_FrontMotorSize input; MtrCtrlFault_HeightHallCnt input; MtrCtrlFault_LengthHallCnt input; MtrCtrlFault_BackHallCnt input; MtrCtrlFault_FrontHallCnt input; HeightSoftStopBufCnt local uint8; LengthSoftStopBufCnt local uint8; BackSoftStopBufCnt local uint8; FrontSoftStopBufCnt local uint8; FALSE parameter; TRUE parameter; D_DrSoftStopDef_B parameter; D_DrSoftStopDef_L parameter; D_DrSoftStopDef_H parameter; D_DrSoftStopDef_F parameter

== stateflow chart APPL_PaFaultDetection/LogicCtrl/AdheAndEffec/SwitchErrorDetection/TimeDiffTs/Chart ==
  (default) -> (junction 3)
  (junction 3) -> (junction 5)
  (junction 5) -> (junction 7) [order 1] : /* 入参比当前大 */
      | [lastTs > Ts]
  (junction 5) -> (junction 13) [order 2] : {OutTs = Ts - lastTs;}
  (junction 7) -> (junction 11) : {OutTs = 0xFFFFFFFF - lastTs + Ts +1;}
  (junction 11) -> (junction 13)
  (junction 13) -> (junction 17)
  data: lastTs input uint32; Ts input uint32; OutTs output uint32
